simulink model "c00017M_harness"  (R2018a)
settings: Solver=ode3  StartTime=0.0  StopTime=10.0  RelTol=1e-3  EnableMultiTasking=on
undefined symbols (not defined in the file): b, DiscIntNeverNeededParam, J, K, L, PosMinimaW3, PosMinimaW4, R, sigbuilder_block
(part 3 of 68)

== system c00017M_harness/Eval134 ==
  In1 : Inport
  In2 : Inport  Port=2
  In3 : Inport  Port=3
  In4 : Inport  Port=4
  Data Type Conversion{,1..3} (4 alike) : DataTypeConversion
  Memory{1..4} (4 alike) : Memory  InitialCondition=1
  MinMax : MinMax  Inputs=4
  MinMax{1..4} (4 alike) : MinMax  Inputs=2
  ROOut{1..4} (4 alike) : RelationalOperator  Operator===  OutDataTypeStr=boolean  RndMeth=Simplest
  Out1 : Outport
  wires:
  Data Type Conversion3/1 -> MinMax4/1
  Data Type Conversion2/1 -> MinMax3/1
  Data Type Conversion1/1 -> MinMax2/1
  Data Type Conversion/1 -> MinMax1/1
  MinMax1/1 -> Memory1/1, MinMax/1
  ROOut4/1 -> Data Type Conversion3/1
  MinMax2/1 -> Memory2/1, MinMax/2
  ROOut1/1 -> Data Type Conversion/1
  Memory2/1 -> MinMax2/2
  Memory4/1 -> MinMax4/2
  Memory3/1 -> MinMax3/2
  ROOut2/1 -> Data Type Conversion1/1
  ROOut3/1 -> Data Type Conversion2/1
  MinMax3/1 -> Memory3/1, MinMax/3
  MinMax4/1 -> Memory4/1, MinMax/4
  Memory1/1 -> MinMax1/2
  [out4] -> ROOut4/2
  In4/1 -> ROOut4/1
  [out2] -> ROOut2/2
  In1/1 -> ROOut1/1
  In2/1 -> ROOut2/1
  [out1] -> ROOut1/2
  In3/1 -> ROOut3/1
  [out3] -> ROOut3/2
  MinMax/1 -> Out1/1

== system c00017M_harness/Eval135 ==
  In1 : Inport
  In2 : Inport  Port=2
  In3 : Inport  Port=3
  In4 : Inport  Port=4
  Data Type Conversion{,1..3} (4 alike) : DataTypeConversion
  Memory{1..4} (4 alike) : Memory  InitialCondition=1
  MinMax : MinMax  Inputs=4
  MinMax{1..4} (4 alike) : MinMax  Inputs=2
  ROOut{1..4} (4 alike) : RelationalOperator  Operator===  OutDataTypeStr=boolean  RndMeth=Simplest
  Out1 : Outport
  wires:
  Data Type Conversion3/1 -> MinMax4/1
  Data Type Conversion2/1 -> MinMax3/1
  Data Type Conversion1/1 -> MinMax2/1
  Data Type Conversion/1 -> MinMax1/1
  MinMax1/1 -> Memory1/1, MinMax/1
  ROOut4/1 -> Data Type Conversion3/1
  MinMax2/1 -> Memory2/1, MinMax/2
  ROOut1/1 -> Data Type Conversion/1
  Memory2/1 -> MinMax2/2
  Memory4/1 -> MinMax4/2
  Memory3/1 -> MinMax3/2
  ROOut2/1 -> Data Type Conversion1/1
  ROOut3/1 -> Data Type Conversion2/1
  MinMax3/1 -> Memory3/1, MinMax/3
  MinMax4/1 -> Memory4/1, MinMax/4
  Memory1/1 -> MinMax1/2
  [out4] -> ROOut4/2
  In4/1 -> ROOut4/1
  [out2] -> ROOut2/2
  In1/1 -> ROOut1/1
  In2/1 -> ROOut2/1
  [out1] -> ROOut1/2
  In3/1 -> ROOut3/1
  [out3] -> ROOut3/2
  MinMax/1 -> Out1/1

== system c00017M_harness/Eval136 ==
  In1 : Inport
  In2 : Inport  Port=2
  In3 : Inport  Port=3
  In4 : Inport  Port=4
  Data Type Conversion{,1..3} (4 alike) : DataTypeConversion
  Memory{1..4} (4 alike) : Memory  InitialCondition=1
  MinMax : MinMax  Inputs=4
  MinMax{1..4} (4 alike) : MinMax  Inputs=2
  ROOut{1..4} (4 alike) : RelationalOperator  Operator===  OutDataTypeStr=boolean  RndMeth=Simplest
  Out1 : Outport
  wires:
  Data Type Conversion3/1 -> MinMax4/1
  Data Type Conversion2/1 -> MinMax3/1
  Data Type Conversion1/1 -> MinMax2/1
  Data Type Conversion/1 -> MinMax1/1
  MinMax1/1 -> Memory1/1, MinMax/1
  ROOut4/1 -> Data Type Conversion3/1
  MinMax2/1 -> Memory2/1, MinMax/2
  ROOut1/1 -> Data Type Conversion/1
  Memory2/1 -> MinMax2/2
  Memory4/1 -> MinMax4/2
  Memory3/1 -> MinMax3/2
  ROOut2/1 -> Data Type Conversion1/1
  ROOut3/1 -> Data Type Conversion2/1
  MinMax3/1 -> Memory3/1, MinMax/3
  MinMax4/1 -> Memory4/1, MinMax/4
  Memory1/1 -> MinMax1/2
  [out4] -> ROOut4/2
  In4/1 -> ROOut4/1
  [out2] -> ROOut2/2
  In1/1 -> ROOut1/1
  In2/1 -> ROOut2/1
  [out1] -> ROOut1/2
  In3/1 -> ROOut3/1
  [out3] -> ROOut3/2
  MinMax/1 -> Out1/1

== system c00017M_harness/Eval137 ==
  In1 : Inport
  In2 : Inport  Port=2
  In3 : Inport  Port=3
  In4 : Inport  Port=4
  Data Type Conversion{,1..3} (4 alike) : DataTypeConversion
  Memory{1..4} (4 alike) : Memory  InitialCondition=1
  MinMax : MinMax  Inputs=4
  MinMax{1..4} (4 alike) : MinMax  Inputs=2
  ROOut{1..4} (4 alike) : RelationalOperator  Operator===  OutDataTypeStr=boolean  RndMeth=Simplest
  Out1 : Outport
  wires:
  Data Type Conversion3/1 -> MinMax4/1
  Data Type Conversion2/1 -> MinMax3/1
  Data Type Conversion1/1 -> MinMax2/1
  Data Type Conversion/1 -> MinMax1/1
  MinMax1/1 -> Memory1/1, MinMax/1
  ROOut4/1 -> Data Type Conversion3/1
  MinMax2/1 -> Memory2/1, MinMax/2
  ROOut1/1 -> Data Type Conversion/1
  Memory2/1 -> MinMax2/2
  Memory4/1 -> MinMax4/2
  Memory3/1 -> MinMax3/2
  ROOut2/1 -> Data Type Conversion1/1
  ROOut3/1 -> Data Type Conversion2/1
  MinMax3/1 -> Memory3/1, MinMax/3
  MinMax4/1 -> Memory4/1, MinMax/4
  Memory1/1 -> MinMax1/2
  [out4] -> ROOut4/2
  In4/1 -> ROOut4/1
  [out2] -> ROOut2/2
  In1/1 -> ROOut1/1
  In2/1 -> ROOut2/1
  [out1] -> ROOut1/2
  In3/1 -> ROOut3/1
  [out3] -> ROOut3/2
  MinMax/1 -> Out1/1

== system c00017M_harness/Eval138 ==
  In1 : Inport
  In2 : Inport  Port=2
  In3 : Inport  Port=3
  In4 : Inport  Port=4
  Data Type Conversion{,1..3} (4 alike) : DataTypeConversion
  Memory{1..4} (4 alike) : Memory  InitialCondition=1
  MinMax : MinMax  Inputs=4
  MinMax{1..4} (4 alike) : MinMax  Inputs=2
  ROOut{1..4} (4 alike) : RelationalOperator  Operator===  OutDataTypeStr=boolean  RndMeth=Simplest
  Out1 : Outport
  wires:
  Data Type Conversion3/1 -> MinMax4/1
  Data Type Conversion2/1 -> MinMax3/1
  Data Type Conversion1/1 -> MinMax2/1
  Data Type Conversion/1 -> MinMax1/1
  MinMax1/1 -> Memory1/1, MinMax/1
  ROOut4/1 -> Data Type Conversion3/1
  MinMax2/1 -> Memory2/1, MinMax/2
  ROOut1/1 -> Data Type Conversion/1
  Memory2/1 -> MinMax2/2
  Memory4/1 -> MinMax4/2
  Memory3/1 -> MinMax3/2
  ROOut2/1 -> Data Type Conversion1/1
  ROOut3/1 -> Data Type Conversion2/1
  MinMax3/1 -> Memory3/1, MinMax/3
  MinMax4/1 -> Memory4/1, MinMax/4
  Memory1/1 -> MinMax1/2
  [out4] -> ROOut4/2
  In4/1 -> ROOut4/1
  [out2] -> ROOut2/2
  In1/1 -> ROOut1/1
  In2/1 -> ROOut2/1
  [out1] -> ROOut1/2
  In3/1 -> ROOut3/1
  [out3] -> ROOut3/2
  MinMax/1 -> Out1/1

== system c00017M_harness/Eval139 ==
  In1 : Inport
  In2 : Inport  Port=2
  In3 : Inport  Port=3
  In4 : Inport  Port=4
  Data Type Conversion{,1..3} (4 alike) : DataTypeConversion
  Memory{1..4} (4 alike) : Memory  InitialCondition=1
  MinMax : MinMax  Inputs=4
  MinMax{1..4} (4 alike) : MinMax  Inputs=2
  ROOut{1..4} (4 alike) : RelationalOperator  Operator===  OutDataTypeStr=boolean  RndMeth=Simplest
  Out1 : Outport
  wires:
  Data Type Conversion3/1 -> MinMax4/1
  Data Type Conversion2/1 -> MinMax3/1
  Data Type Conversion1/1 -> MinMax2/1
  Data Type Conversion/1 -> MinMax1/1
  MinMax1/1 -> Memory1/1, MinMax/1
  ROOut4/1 -> Data Type Conversion3/1
  MinMax2/1 -> Memory2/1, MinMax/2
  ROOut1/1 -> Data Type Conversion/1
  Memory2/1 -> MinMax2/2
  Memory4/1 -> MinMax4/2
  Memory3/1 -> MinMax3/2
  ROOut2/1 -> Data Type Conversion1/1
  ROOut3/1 -> Data Type Conversion2/1
  MinMax3/1 -> Memory3/1, MinMax/3
  MinMax4/1 -> Memory4/1, MinMax/4
  Memory1/1 -> MinMax1/2
  [out4] -> ROOut4/2
  In4/1 -> ROOut4/1
  [out2] -> ROOut2/2
  In1/1 -> ROOut1/1
  In2/1 -> ROOut2/1
  [out1] -> ROOut1/2
  In3/1 -> ROOut3/1
  [out3] -> ROOut3/2
  MinMax/1 -> Out1/1

== system c00017M_harness/Eval14 ==
  In1 : Inport
  In2 : Inport  Port=2
  In3 : Inport  Port=3
  In4 : Inport  Port=4
  Data Type Conversion{,1..3} (4 alike) : DataTypeConversion
  Memory{1..4} (4 alike) : Memory  InitialCondition=1
  MinMax : MinMax  Inputs=4
  MinMax{1..4} (4 alike) : MinMax  Inputs=2
  ROOut{1..4} (4 alike) : RelationalOperator  Operator===  OutDataTypeStr=boolean  RndMeth=Simplest
  Out1 : Outport
  wires:
  Data Type Conversion3/1 -> MinMax4/1
  Data Type Conversion2/1 -> MinMax3/1
  Data Type Conversion1/1 -> MinMax2/1
  Data Type Conversion/1 -> MinMax1/1
  MinMax1/1 -> Memory1/1, MinMax/1
  ROOut4/1 -> Data Type Conversion3/1
  MinMax2/1 -> Memory2/1, MinMax/2
  ROOut1/1 -> Data Type Conversion/1
  Memory2/1 -> MinMax2/2
  Memory4/1 -> MinMax4/2
  Memory3/1 -> MinMax3/2
  ROOut2/1 -> Data Type Conversion1/1
  ROOut3/1 -> Data Type Conversion2/1
  MinMax3/1 -> Memory3/1, MinMax/3
  MinMax4/1 -> Memory4/1, MinMax/4
  Memory1/1 -> MinMax1/2
  [out4] -> ROOut4/2
  In4/1 -> ROOut4/1
  [out2] -> ROOut2/2
  In1/1 -> ROOut1/1
  In2/1 -> ROOut2/1
  [out1] -> ROOut1/2
  In3/1 -> ROOut3/1
  [out3] -> ROOut3/2
  MinMax/1 -> Out1/1

== system c00017M_harness/Eval140 ==
  In1 : Inport
  In2 : Inport  Port=2
  In3 : Inport  Port=3
  In4 : Inport  Port=4
  Data Type Conversion{,1..3} (4 alike) : DataTypeConversion
  Memory{1..4} (4 alike) : Memory  InitialCondition=1
  MinMax : MinMax  Inputs=4
  MinMax{1..4} (4 alike) : MinMax  Inputs=2
  ROOut{1..4} (4 alike) : RelationalOperator  Operator===  OutDataTypeStr=boolean  RndMeth=Simplest
  Out1 : Outport
  wires:
  Data Type Conversion3/1 -> MinMax4/1
  Data Type Conversion2/1 -> MinMax3/1
  Data Type Conversion1/1 -> MinMax2/1
  Data Type Conversion/1 -> MinMax1/1
  MinMax1/1 -> Memory1/1, MinMax/1
  ROOut4/1 -> Data Type Conversion3/1
  MinMax2/1 -> Memory2/1, MinMax/2
  ROOut1/1 -> Data Type Conversion/1
  Memory2/1 -> MinMax2/2
  Memory4/1 -> MinMax4/2
  Memory3/1 -> MinMax3/2
  ROOut2/1 -> Data Type Conversion1/1
  ROOut3/1 -> Data Type Conversion2/1
  MinMax3/1 -> Memory3/1, MinMax/3
  MinMax4/1 -> Memory4/1, MinMax/4
  Memory1/1 -> MinMax1/2
  [out4] -> ROOut4/2
  In4/1 -> ROOut4/1
  [out2] -> ROOut2/2
  In1/1 -> ROOut1/1
  In2/1 -> ROOut2/1
  [out1] -> ROOut1/2
  In3/1 -> ROOut3/1
  [out3] -> ROOut3/2
  MinMax/1 -> Out1/1

== system c00017M_harness/Eval141 ==
  In1 : Inport
  In2 : Inport  Port=2
  In3 : Inport  Port=3
  In4 : Inport  Port=4
  Data Type Conversion{,1..3} (4 alike) : DataTypeConversion
  Memory{1..4} (4 alike) : Memory  InitialCondition=1
  MinMax : MinMax  Inputs=4
  MinMax{1..4} (4 alike) : MinMax  Inputs=2
  ROOut{1..4} (4 alike) : RelationalOperator  Operator===  OutDataTypeStr=boolean  RndMeth=Simplest
  Out1 : Outport
  wires:
  Data Type Conversion3/1 -> MinMax4/1
  Data Type Conversion2/1 -> MinMax3/1
  Data Type Conversion1/1 -> MinMax2/1
  Data Type Conversion/1 -> MinMax1/1
  MinMax1/1 -> Memory1/1, MinMax/1
  ROOut4/1 -> Data Type Conversion3/1
  MinMax2/1 -> Memory2/1, MinMax/2
  ROOut1/1 -> Data Type Conversion/1
  Memory2/1 -> MinMax2/2
  Memory4/1 -> MinMax4/2
  Memory3/1 -> MinMax3/2
  ROOut2/1 -> Data Type Conversion1/1
  ROOut3/1 -> Data Type Conversion2/1
  MinMax3/1 -> Memory3/1, MinMax/3
  MinMax4/1 -> Memory4/1, MinMax/4
  Memory1/1 -> MinMax1/2
  [out4] -> ROOut4/2
  In4/1 -> ROOut4/1
  [out2] -> ROOut2/2
  In1/1 -> ROOut1/1
  In2/1 -> ROOut2/1
  [out1] -> ROOut1/2
  In3/1 -> ROOut3/1
  [out3] -> ROOut3/2
  MinMax/1 -> Out1/1

== system c00017M_harness/Eval142 ==
  In1 : Inport
  In2 : Inport  Port=2
  In3 : Inport  Port=3
  In4 : Inport  Port=4
  Data Type Conversion{,1..3} (4 alike) : DataTypeConversion
  Memory{1..4} (4 alike) : Memory  InitialCondition=1
  MinMax : MinMax  Inputs=4
  MinMax{1..4} (4 alike) : MinMax  Inputs=2
  ROOut{1..4} (4 alike) : RelationalOperator  Operator===  OutDataTypeStr=boolean  RndMeth=Simplest
  Out1 : Outport
  wires:
  Data Type Conversion3/1 -> MinMax4/1
  Data Type Conversion2/1 -> MinMax3/1
  Data Type Conversion1/1 -> MinMax2/1
  Data Type Conversion/1 -> MinMax1/1
  MinMax1/1 -> Memory1/1, MinMax/1
  ROOut4/1 -> Data Type Conversion3/1
  MinMax2/1 -> Memory2/1, MinMax/2
  ROOut1/1 -> Data Type Conversion/1
  Memory2/1 -> MinMax2/2
  Memory4/1 -> MinMax4/2
  Memory3/1 -> MinMax3/2
  ROOut2/1 -> Data Type Conversion1/1
  ROOut3/1 -> Data Type Conversion2/1
  MinMax3/1 -> Memory3/1, MinMax/3
  MinMax4/1 -> Memory4/1, MinMax/4
  Memory1/1 -> MinMax1/2
  [out4] -> ROOut4/2
  In4/1 -> ROOut4/1
  [out2] -> ROOut2/2
  In1/1 -> ROOut1/1
  In2/1 -> ROOut2/1
  [out1] -> ROOut1/2
  In3/1 -> ROOut3/1
  [out3] -> ROOut3/2
  MinMax/1 -> Out1/1

== system c00017M_harness/Eval143 ==
  In1 : Inport
  In2 : Inport  Port=2
  In3 : Inport  Port=3
  In4 : Inport  Port=4
  Data Type Conversion{,1..3} (4 alike) : DataTypeConversion
  Memory{1..4} (4 alike) : Memory  InitialCondition=1
  MinMax : MinMax  Inputs=4
  MinMax{1..4} (4 alike) : MinMax  Inputs=2
  ROOut{1..4} (4 alike) : RelationalOperator  Operator===  OutDataTypeStr=boolean  RndMeth=Simplest
  Out1 : Outport
  wires:
  Data Type Conversion3/1 -> MinMax4/1
  Data Type Conversion2/1 -> MinMax3/1
  Data Type Conversion1/1 -> MinMax2/1
  Data Type Conversion/1 -> MinMax1/1
  MinMax1/1 -> Memory1/1, MinMax/1
  ROOut4/1 -> Data Type Conversion3/1
  MinMax2/1 -> Memory2/1, MinMax/2
  ROOut1/1 -> Data Type Conversion/1
  Memory2/1 -> MinMax2/2
  Memory4/1 -> MinMax4/2
  Memory3/1 -> MinMax3/2
  ROOut2/1 -> Data Type Conversion1/1
  ROOut3/1 -> Data Type Conversion2/1
  MinMax3/1 -> Memory3/1, MinMax/3
  MinMax4/1 -> Memory4/1, MinMax/4
  Memory1/1 -> MinMax1/2
  [out4] -> ROOut4/2
  In4/1 -> ROOut4/1
  [out2] -> ROOut2/2
  In1/1 -> ROOut1/1
  In2/1 -> ROOut2/1
  [out1] -> ROOut1/2
  In3/1 -> ROOut3/1
  [out3] -> ROOut3/2
  MinMax/1 -> Out1/1

== system c00017M_harness/Eval144 ==
  In1 : Inport
  In2 : Inport  Port=2
  In3 : Inport  Port=3
  In4 : Inport  Port=4
  Data Type Conversion{,1..3} (4 alike) : DataTypeConversion
  Memory{1..4} (4 alike) : Memory  InitialCondition=1
  MinMax : MinMax  Inputs=4
  MinMax{1..4} (4 alike) : MinMax  Inputs=2
  ROOut{1..4} (4 alike) : RelationalOperator  Operator===  OutDataTypeStr=boolean  RndMeth=Simplest
  Out1 : Outport
  wires:
  Data Type Conversion3/1 -> MinMax4/1
  Data Type Conversion2/1 -> MinMax3/1
  Data Type Conversion1/1 -> MinMax2/1
  Data Type Conversion/1 -> MinMax1/1
  MinMax1/1 -> Memory1/1, MinMax/1
  ROOut4/1 -> Data Type Conversion3/1
  MinMax2/1 -> Memory2/1, MinMax/2
  ROOut1/1 -> Data Type Conversion/1
  Memory2/1 -> MinMax2/2
  Memory4/1 -> MinMax4/2
  Memory3/1 -> MinMax3/2
  ROOut2/1 -> Data Type Conversion1/1
  ROOut3/1 -> Data Type Conversion2/1
  MinMax3/1 -> Memory3/1, MinMax/3
  MinMax4/1 -> Memory4/1, MinMax/4
  Memory1/1 -> MinMax1/2
  [out4] -> ROOut4/2
  In4/1 -> ROOut4/1
  [out2] -> ROOut2/2
  In1/1 -> ROOut1/1
  In2/1 -> ROOut2/1
  [out1] -> ROOut1/2
  In3/1 -> ROOut3/1
  [out3] -> ROOut3/2
  MinMax/1 -> Out1/1

== system c00017M_harness/Eval145 ==
  In1 : Inport
  In2 : Inport  Port=2
  In3 : Inport  Port=3
  In4 : Inport  Port=4
  Data Type Conversion{,1..3} (4 alike) : DataTypeConversion
  Memory{1..4} (4 alike) : Memory  InitialCondition=1
  MinMax : MinMax  Inputs=4
  MinMax{1..4} (4 alike) : MinMax  Inputs=2
  ROOut{1..4} (4 alike) : RelationalOperator  Operator===  OutDataTypeStr=boolean  RndMeth=Simplest
  Out1 : Outport
  wires:
  Data Type Conversion3/1 -> MinMax4/1
  Data Type Conversion2/1 -> MinMax3/1
  Data Type Conversion1/1 -> MinMax2/1
  Data Type Conversion/1 -> MinMax1/1
  MinMax1/1 -> Memory1/1, MinMax/1
  ROOut4/1 -> Data Type Conversion3/1
  MinMax2/1 -> Memory2/1, MinMax/2
  ROOut1/1 -> Data Type Conversion/1
  Memory2/1 -> MinMax2/2
  Memory4/1 -> MinMax4/2
  Memory3/1 -> MinMax3/2
  ROOut2/1 -> Data Type Conversion1/1
  ROOut3/1 -> Data Type Conversion2/1
  MinMax3/1 -> Memory3/1, MinMax/3
  MinMax4/1 -> Memory4/1, MinMax/4
  Memory1/1 -> MinMax1/2
  [out4] -> ROOut4/2
  In4/1 -> ROOut4/1
  [out2] -> ROOut2/2
  In1/1 -> ROOut1/1
  In2/1 -> ROOut2/1
  [out1] -> ROOut1/2
  In3/1 -> ROOut3/1
  [out3] -> ROOut3/2
  MinMax/1 -> Out1/1

== system c00017M_harness/Eval146 ==
  In1 : Inport
  In2 : Inport  Port=2
  In3 : Inport  Port=3
  In4 : Inport  Port=4
  Data Type Conversion{,1..3} (4 alike) : DataTypeConversion
  Memory{1..4} (4 alike) : Memory  InitialCondition=1
  MinMax : MinMax  Inputs=4
  MinMax{1..4} (4 alike) : MinMax  Inputs=2
  ROOut{1..4} (4 alike) : RelationalOperator  Operator===  OutDataTypeStr=boolean  RndMeth=Simplest
  Out1 : Outport
  wires:
  Data Type Conversion3/1 -> MinMax4/1
  Data Type Conversion2/1 -> MinMax3/1
  Data Type Conversion1/1 -> MinMax2/1
  Data Type Conversion/1 -> MinMax1/1
  MinMax1/1 -> Memory1/1, MinMax/1
  ROOut4/1 -> Data Type Conversion3/1
  MinMax2/1 -> Memory2/1, MinMax/2
  ROOut1/1 -> Data Type Conversion/1
  Memory2/1 -> MinMax2/2
  Memory4/1 -> MinMax4/2
  Memory3/1 -> MinMax3/2
  ROOut2/1 -> Data Type Conversion1/1
  ROOut3/1 -> Data Type Conversion2/1
  MinMax3/1 -> Memory3/1, MinMax/3
  MinMax4/1 -> Memory4/1, MinMax/4
  Memory1/1 -> MinMax1/2
  [out4] -> ROOut4/2
  In4/1 -> ROOut4/1
  [out2] -> ROOut2/2
  In1/1 -> ROOut1/1
  In2/1 -> ROOut2/1
  [out1] -> ROOut1/2
  In3/1 -> ROOut3/1
  [out3] -> ROOut3/2
  MinMax/1 -> Out1/1

== system c00017M_harness/Eval147 ==
  In1 : Inport
  In2 : Inport  Port=2
  In3 : Inport  Port=3
  In4 : Inport  Port=4
  Data Type Conversion{,1..3} (4 alike) : DataTypeConversion
  Memory{1..4} (4 alike) : Memory  InitialCondition=1
  MinMax : MinMax  Inputs=4
  MinMax{1..4} (4 alike) : MinMax  Inputs=2
  ROOut{1..4} (4 alike) : RelationalOperator  Operator===  OutDataTypeStr=boolean  RndMeth=Simplest
  Out1 : Outport
  wires:
  Data Type Conversion3/1 -> MinMax4/1
  Data Type Conversion2/1 -> MinMax3/1
  Data Type Conversion1/1 -> MinMax2/1
  Data Type Conversion/1 -> MinMax1/1
  MinMax1/1 -> Memory1/1, MinMax/1
  ROOut4/1 -> Data Type Conversion3/1
  MinMax2/1 -> Memory2/1, MinMax/2
  ROOut1/1 -> Data Type Conversion/1
  Memory2/1 -> MinMax2/2
  Memory4/1 -> MinMax4/2
  Memory3/1 -> MinMax3/2
  ROOut2/1 -> Data Type Conversion1/1
  ROOut3/1 -> Data Type Conversion2/1
  MinMax3/1 -> Memory3/1, MinMax/3
  MinMax4/1 -> Memory4/1, MinMax/4
  Memory1/1 -> MinMax1/2
  [out4] -> ROOut4/2
  In4/1 -> ROOut4/1
  [out2] -> ROOut2/2
  In1/1 -> ROOut1/1
  In2/1 -> ROOut2/1
  [out1] -> ROOut1/2
  In3/1 -> ROOut3/1
  [out3] -> ROOut3/2
  MinMax/1 -> Out1/1

== system c00017M_harness/Eval148 ==
  In1 : Inport
  In2 : Inport  Port=2
  In3 : Inport  Port=3
  In4 : Inport  Port=4
  Data Type Conversion{,1..3} (4 alike) : DataTypeConversion
  Memory{1..4} (4 alike) : Memory  InitialCondition=1
  MinMax : MinMax  Inputs=4
  MinMax{1..4} (4 alike) : MinMax  Inputs=2
  ROOut{1..4} (4 alike) : RelationalOperator  Operator===  OutDataTypeStr=boolean  RndMeth=Simplest
  Out1 : Outport
  wires:
  Data Type Conversion3/1 -> MinMax4/1
  Data Type Conversion2/1 -> MinMax3/1
  Data Type Conversion1/1 -> MinMax2/1
  Data Type Conversion/1 -> MinMax1/1
  MinMax1/1 -> Memory1/1, MinMax/1
  ROOut4/1 -> Data Type Conversion3/1
  MinMax2/1 -> Memory2/1, MinMax/2
  ROOut1/1 -> Data Type Conversion/1
  Memory2/1 -> MinMax2/2
  Memory4/1 -> MinMax4/2
  Memory3/1 -> MinMax3/2
  ROOut2/1 -> Data Type Conversion1/1
  ROOut3/1 -> Data Type Conversion2/1
  MinMax3/1 -> Memory3/1, MinMax/3
  MinMax4/1 -> Memory4/1, MinMax/4
  Memory1/1 -> MinMax1/2
  [out4] -> ROOut4/2
  In4/1 -> ROOut4/1
  [out2] -> ROOut2/2
  In1/1 -> ROOut1/1
  In2/1 -> ROOut2/1
  [out1] -> ROOut1/2
  In3/1 -> ROOut3/1
  [out3] -> ROOut3/2
  MinMax/1 -> Out1/1

== system c00017M_harness/Eval149 ==
  In1 : Inport
  In2 : Inport  Port=2
  In3 : Inport  Port=3
  In4 : Inport  Port=4
  Data Type Conversion{,1..3} (4 alike) : DataTypeConversion
  Memory{1..4} (4 alike) : Memory  InitialCondition=1
  MinMax : MinMax  Inputs=4
  MinMax{1..4} (4 alike) : MinMax  Inputs=2
  ROOut{1..4} (4 alike) : RelationalOperator  Operator===  OutDataTypeStr=boolean  RndMeth=Simplest
  Out1 : Outport
  wires:
  Data Type Conversion3/1 -> MinMax4/1
  Data Type Conversion2/1 -> MinMax3/1
  Data Type Conversion1/1 -> MinMax2/1
  Data Type Conversion/1 -> MinMax1/1
  MinMax1/1 -> Memory1/1, MinMax/1
  ROOut4/1 -> Data Type Conversion3/1
  MinMax2/1 -> Memory2/1, MinMax/2
  ROOut1/1 -> Data Type Conversion/1
  Memory2/1 -> MinMax2/2
  Memory4/1 -> MinMax4/2
  Memory3/1 -> MinMax3/2
  ROOut2/1 -> Data Type Conversion1/1
  ROOut3/1 -> Data Type Conversion2/1
  MinMax3/1 -> Memory3/1, MinMax/3
  MinMax4/1 -> Memory4/1, MinMax/4
  Memory1/1 -> MinMax1/2
  [out4] -> ROOut4/2
  In4/1 -> ROOut4/1
  [out2] -> ROOut2/2
  In1/1 -> ROOut1/1
  In2/1 -> ROOut2/1
  [out1] -> ROOut1/2
  In3/1 -> ROOut3/1
  [out3] -> ROOut3/2
  MinMax/1 -> Out1/1

== system c00017M_harness/Eval15 ==
  In1 : Inport
  In2 : Inport  Port=2
  In3 : Inport  Port=3
  In4 : Inport  Port=4
  Data Type Conversion{,1..3} (4 alike) : DataTypeConversion
  Memory{1..4} (4 alike) : Memory  InitialCondition=1
  MinMax : MinMax  Inputs=4
  MinMax{1..4} (4 alike) : MinMax  Inputs=2
  ROOut{1..4} (4 alike) : RelationalOperator  Operator===  OutDataTypeStr=boolean  RndMeth=Simplest
  Out1 : Outport
  wires:
  Data Type Conversion3/1 -> MinMax4/1
  Data Type Conversion2/1 -> MinMax3/1
  Data Type Conversion1/1 -> MinMax2/1
  Data Type Conversion/1 -> MinMax1/1
  MinMax1/1 -> Memory1/1, MinMax/1
  ROOut4/1 -> Data Type Conversion3/1
  MinMax2/1 -> Memory2/1, MinMax/2
  ROOut1/1 -> Data Type Conversion/1
  Memory2/1 -> MinMax2/2
  Memory4/1 -> MinMax4/2
  Memory3/1 -> MinMax3/2
  ROOut2/1 -> Data Type Conversion1/1
  ROOut3/1 -> Data Type Conversion2/1
  MinMax3/1 -> Memory3/1, MinMax/3
  MinMax4/1 -> Memory4/1, MinMax/4
  Memory1/1 -> MinMax1/2
  [out4] -> ROOut4/2
  In4/1 -> ROOut4/1
  [out2] -> ROOut2/2
  In1/1 -> ROOut1/1
  In2/1 -> ROOut2/1
  [out1] -> ROOut1/2
  In3/1 -> ROOut3/1
  [out3] -> ROOut3/2
  MinMax/1 -> Out1/1

== system c00017M_harness/Eval150 ==
  In1 : Inport
  In2 : Inport  Port=2
  In3 : Inport  Port=3
  In4 : Inport  Port=4
  Data Type Conversion{,1..3} (4 alike) : DataTypeConversion
  Memory{1..4} (4 alike) : Memory  InitialCondition=1
  MinMax : MinMax  Inputs=4
  MinMax{1..4} (4 alike) : MinMax  Inputs=2
  ROOut{1..4} (4 alike) : RelationalOperator  Operator===  OutDataTypeStr=boolean  RndMeth=Simplest
  Out1 : Outport
  wires:
  Data Type Conversion3/1 -> MinMax4/1
  Data Type Conversion2/1 -> MinMax3/1
  Data Type Conversion1/1 -> MinMax2/1
  Data Type Conversion/1 -> MinMax1/1
  MinMax1/1 -> Memory1/1, MinMax/1
  ROOut4/1 -> Data Type Conversion3/1
  MinMax2/1 -> Memory2/1, MinMax/2
  ROOut1/1 -> Data Type Conversion/1
  Memory2/1 -> MinMax2/2
  Memory4/1 -> MinMax4/2
  Memory3/1 -> MinMax3/2
  ROOut2/1 -> Data Type Conversion1/1
  ROOut3/1 -> Data Type Conversion2/1
  MinMax3/1 -> Memory3/1, MinMax/3
  MinMax4/1 -> Memory4/1, MinMax/4
  Memory1/1 -> MinMax1/2
  [out4] -> ROOut4/2
  In4/1 -> ROOut4/1
  [out2] -> ROOut2/2
  In1/1 -> ROOut1/1
  In2/1 -> ROOut2/1
  [out1] -> ROOut1/2
  In3/1 -> ROOut3/1
  [out3] -> ROOut3/2
  MinMax/1 -> Out1/1

== system c00017M_harness/Eval151 ==
  In1 : Inport
  In2 : Inport  Port=2
  In3 : Inport  Port=3
  In4 : Inport  Port=4
  Data Type Conversion{,1..3} (4 alike) : DataTypeConversion
  Memory{1..4} (4 alike) : Memory  InitialCondition=1
  MinMax : MinMax  Inputs=4
  MinMax{1..4} (4 alike) : MinMax  Inputs=2
  ROOut{1..4} (4 alike) : RelationalOperator  Operator===  OutDataTypeStr=boolean  RndMeth=Simplest
  Out1 : Outport
  wires:
  Data Type Conversion3/1 -> MinMax4/1
  Data Type Conversion2/1 -> MinMax3/1
  Data Type Conversion1/1 -> MinMax2/1
  Data Type Conversion/1 -> MinMax1/1
  MinMax1/1 -> Memory1/1, MinMax/1
  ROOut4/1 -> Data Type Conversion3/1
  MinMax2/1 -> Memory2/1, MinMax/2
  ROOut1/1 -> Data Type Conversion/1
  Memory2/1 -> MinMax2/2
  Memory4/1 -> MinMax4/2
  Memory3/1 -> MinMax3/2
  ROOut2/1 -> Data Type Conversion1/1
  ROOut3/1 -> Data Type Conversion2/1
  MinMax3/1 -> Memory3/1, MinMax/3
  MinMax4/1 -> Memory4/1, MinMax/4
  Memory1/1 -> MinMax1/2
  [out4] -> ROOut4/2
  In4/1 -> ROOut4/1
  [out2] -> ROOut2/2
  In1/1 -> ROOut1/1
  In2/1 -> ROOut2/1
  [out1] -> ROOut1/2
  In3/1 -> ROOut3/1
  [out3] -> ROOut3/2
  MinMax/1 -> Out1/1

== system c00017M_harness/Eval152 ==
  In1 : Inport
  In2 : Inport  Port=2
  In3 : Inport  Port=3
  In4 : Inport  Port=4
  Data Type Conversion{,1..3} (4 alike) : DataTypeConversion
  Memory{1..4} (4 alike) : Memory  InitialCondition=1
  MinMax : MinMax  Inputs=4
  MinMax{1..4} (4 alike) : MinMax  Inputs=2
  ROOut{1..4} (4 alike) : RelationalOperator  Operator===  OutDataTypeStr=boolean  RndMeth=Simplest
  Out1 : Outport
  wires:
  Data Type Conversion3/1 -> MinMax4/1
  Data Type Conversion2/1 -> MinMax3/1
  Data Type Conversion1/1 -> MinMax2/1
  Data Type Conversion/1 -> MinMax1/1
  MinMax1/1 -> Memory1/1, MinMax/1
  ROOut4/1 -> Data Type Conversion3/1
  MinMax2/1 -> Memory2/1, MinMax/2
  ROOut1/1 -> Data Type Conversion/1
  Memory2/1 -> MinMax2/2
  Memory4/1 -> MinMax4/2
  Memory3/1 -> MinMax3/2
  ROOut2/1 -> Data Type Conversion1/1
  ROOut3/1 -> Data Type Conversion2/1
  MinMax3/1 -> Memory3/1, MinMax/3
  MinMax4/1 -> Memory4/1, MinMax/4
  Memory1/1 -> MinMax1/2
  [out4] -> ROOut4/2
  In4/1 -> ROOut4/1
  [out2] -> ROOut2/2
  In1/1 -> ROOut1/1
  In2/1 -> ROOut2/1
  [out1] -> ROOut1/2
  In3/1 -> ROOut3/1
  [out3] -> ROOut3/2
  MinMax/1 -> Out1/1

== system c00017M_harness/Eval153 ==
  In1 : Inport
  In2 : Inport  Port=2
  In3 : Inport  Port=3
  In4 : Inport  Port=4
  Data Type Conversion{,1..3} (4 alike) : DataTypeConversion
  Memory{1..4} (4 alike) : Memory  InitialCondition=1
  MinMax : MinMax  Inputs=4
  MinMax{1..4} (4 alike) : MinMax  Inputs=2
  ROOut{1..4} (4 alike) : RelationalOperator  Operator===  OutDataTypeStr=boolean  RndMeth=Simplest
  Out1 : Outport
  wires:
  Data Type Conversion3/1 -> MinMax4/1
  Data Type Conversion2/1 -> MinMax3/1
  Data Type Conversion1/1 -> MinMax2/1
  Data Type Conversion/1 -> MinMax1/1
  MinMax1/1 -> Memory1/1, MinMax/1
  ROOut4/1 -> Data Type Conversion3/1
  MinMax2/1 -> Memory2/1, MinMax/2
  ROOut1/1 -> Data Type Conversion/1
  Memory2/1 -> MinMax2/2
  Memory4/1 -> MinMax4/2
  Memory3/1 -> MinMax3/2
  ROOut2/1 -> Data Type Conversion1/1
  ROOut3/1 -> Data Type Conversion2/1
  MinMax3/1 -> Memory3/1, MinMax/3
  MinMax4/1 -> Memory4/1, MinMax/4
  Memory1/1 -> MinMax1/2
  [out4] -> ROOut4/2
  In4/1 -> ROOut4/1
  [out2] -> ROOut2/2
  In1/1 -> ROOut1/1
  In2/1 -> ROOut2/1
  [out1] -> ROOut1/2
  In3/1 -> ROOut3/1
  [out3] -> ROOut3/2
  MinMax/1 -> Out1/1

== system c00017M_harness/Eval154 ==
  In1 : Inport
  In2 : Inport  Port=2
  In3 : Inport  Port=3
  In4 : Inport  Port=4
  Data Type Conversion{,1..3} (4 alike) : DataTypeConversion
  Memory{1..4} (4 alike) : Memory  InitialCondition=1
  MinMax : MinMax  Inputs=4
  MinMax{1..4} (4 alike) : MinMax  Inputs=2
  ROOut{1..4} (4 alike) : RelationalOperator  Operator===  OutDataTypeStr=boolean  RndMeth=Simplest
  Out1 : Outport
  wires:
  Data Type Conversion3/1 -> MinMax4/1
  Data Type Conversion2/1 -> MinMax3/1
  Data Type Conversion1/1 -> MinMax2/1
  Data Type Conversion/1 -> MinMax1/1
  MinMax1/1 -> Memory1/1, MinMax/1
  ROOut4/1 -> Data Type Conversion3/1
  MinMax2/1 -> Memory2/1, MinMax/2
  ROOut1/1 -> Data Type Conversion/1
  Memory2/1 -> MinMax2/2
  Memory4/1 -> MinMax4/2
  Memory3/1 -> MinMax3/2
  ROOut2/1 -> Data Type Conversion1/1
  ROOut3/1 -> Data Type Conversion2/1
  MinMax3/1 -> Memory3/1, MinMax/3
  MinMax4/1 -> Memory4/1, MinMax/4
  Memory1/1 -> MinMax1/2
  [out4] -> ROOut4/2
  In4/1 -> ROOut4/1
  [out2] -> ROOut2/2
  In1/1 -> ROOut1/1
  In2/1 -> ROOut2/1
  [out1] -> ROOut1/2
  In3/1 -> ROOut3/1
  [out3] -> ROOut3/2
  MinMax/1 -> Out1/1

== system c00017M_harness/Eval155 ==
  In1 : Inport
  In2 : Inport  Port=2
  In3 : Inport  Port=3
  In4 : Inport  Port=4
  Data Type Conversion{,1..3} (4 alike) : DataTypeConversion
  Memory{1..4} (4 alike) : Memory  InitialCondition=1
  MinMax : MinMax  Inputs=4
  MinMax{1..4} (4 alike) : MinMax  Inputs=2
  ROOut{1..4} (4 alike) : RelationalOperator  Operator===  OutDataTypeStr=boolean  RndMeth=Simplest
  Out1 : Outport
  wires:
  Data Type Conversion3/1 -> MinMax4/1
  Data Type Conversion2/1 -> MinMax3/1
  Data Type Conversion1/1 -> MinMax2/1
  Data Type Conversion/1 -> MinMax1/1
  MinMax1/1 -> Memory1/1, MinMax/1
  ROOut4/1 -> Data Type Conversion3/1
  MinMax2/1 -> Memory2/1, MinMax/2
  ROOut1/1 -> Data Type Conversion/1
  Memory2/1 -> MinMax2/2
  Memory4/1 -> MinMax4/2
  Memory3/1 -> MinMax3/2
  ROOut2/1 -> Data Type Conversion1/1
  ROOut3/1 -> Data Type Conversion2/1
  MinMax3/1 -> Memory3/1, MinMax/3
  MinMax4/1 -> Memory4/1, MinMax/4
  Memory1/1 -> MinMax1/2
  [out4] -> ROOut4/2
  In4/1 -> ROOut4/1
  [out2] -> ROOut2/2
  In1/1 -> ROOut1/1
  In2/1 -> ROOut2/1
  [out1] -> ROOut1/2
  In3/1 -> ROOut3/1
  [out3] -> ROOut3/2
  MinMax/1 -> Out1/1

== system c00017M_harness/Eval156 ==
  In1 : Inport
  In2 : Inport  Port=2
  In3 : Inport  Port=3
  In4 : Inport  Port=4
  Data Type Conversion{,1..3} (4 alike) : DataTypeConversion
  Memory{1..4} (4 alike) : Memory  InitialCondition=1
  MinMax : MinMax  Inputs=4
  MinMax{1..4} (4 alike) : MinMax  Inputs=2
  ROOut{1..4} (4 alike) : RelationalOperator  Operator===  OutDataTypeStr=boolean  RndMeth=Simplest
  Out1 : Outport
  wires:
  Data Type Conversion3/1 -> MinMax4/1
  Data Type Conversion2/1 -> MinMax3/1
  Data Type Conversion1/1 -> MinMax2/1
  Data Type Conversion/1 -> MinMax1/1
  MinMax1/1 -> Memory1/1, MinMax/1
  ROOut4/1 -> Data Type Conversion3/1
  MinMax2/1 -> Memory2/1, MinMax/2
  ROOut1/1 -> Data Type Conversion/1
  Memory2/1 -> MinMax2/2
  Memory4/1 -> MinMax4/2
  Memory3/1 -> MinMax3/2
  ROOut2/1 -> Data Type Conversion1/1
  ROOut3/1 -> Data Type Conversion2/1
  MinMax3/1 -> Memory3/1, MinMax/3
  MinMax4/1 -> Memory4/1, MinMax/4
  Memory1/1 -> MinMax1/2
  [out4] -> ROOut4/2
  In4/1 -> ROOut4/1
  [out2] -> ROOut2/2
  In1/1 -> ROOut1/1
  In2/1 -> ROOut2/1
  [out1] -> ROOut1/2
  In3/1 -> ROOut3/1
  [out3] -> ROOut3/2
  MinMax/1 -> Out1/1

== system c00017M_harness/Eval157 ==
  In1 : Inport
  In2 : Inport  Port=2
  In3 : Inport  Port=3
  In4 : Inport  Port=4
  Data Type Conversion{,1..3} (4 alike) : DataTypeConversion
  Memory{1..4} (4 alike) : Memory  InitialCondition=1
  MinMax : MinMax  Inputs=4
  MinMax{1..4} (4 alike) : MinMax  Inputs=2
  ROOut{1..4} (4 alike) : RelationalOperator  Operator===  OutDataTypeStr=boolean  RndMeth=Simplest
  Out1 : Outport
  wires:
  Data Type Conversion3/1 -> MinMax4/1
  Data Type Conversion2/1 -> MinMax3/1
  Data Type Conversion1/1 -> MinMax2/1
  Data Type Conversion/1 -> MinMax1/1
  MinMax1/1 -> Memory1/1, MinMax/1
  ROOut4/1 -> Data Type Conversion3/1
  MinMax2/1 -> Memory2/1, MinMax/2
  ROOut1/1 -> Data Type Conversion/1
  Memory2/1 -> MinMax2/2
  Memory4/1 -> MinMax4/2
  Memory3/1 -> MinMax3/2
  ROOut2/1 -> Data Type Conversion1/1
  ROOut3/1 -> Data Type Conversion2/1
  MinMax3/1 -> Memory3/1, MinMax/3
  MinMax4/1 -> Memory4/1, MinMax/4
  Memory1/1 -> MinMax1/2
  [out4] -> ROOut4/2
  In4/1 -> ROOut4/1
  [out2] -> ROOut2/2
  In1/1 -> ROOut1/1
  In2/1 -> ROOut2/1
  [out1] -> ROOut1/2
  In3/1 -> ROOut3/1
  [out3] -> ROOut3/2
  MinMax/1 -> Out1/1

== system c00017M_harness/Eval158 ==
  In1 : Inport
  In2 : Inport  Port=2
  In3 : Inport  Port=3
  In4 : Inport  Port=4
  Data Type Conversion{,1..3} (4 alike) : DataTypeConversion
  Memory{1..4} (4 alike) : Memory  InitialCondition=1
  MinMax : MinMax  Inputs=4
  MinMax{1..4} (4 alike) : MinMax  Inputs=2
  ROOut{1..4} (4 alike) : RelationalOperator  Operator===  OutDataTypeStr=boolean  RndMeth=Simplest
  Out1 : Outport
  wires:
  Data Type Conversion3/1 -> MinMax4/1
  Data Type Conversion2/1 -> MinMax3/1
  Data Type Conversion1/1 -> MinMax2/1
  Data Type Conversion/1 -> MinMax1/1
  MinMax1/1 -> Memory1/1, MinMax/1
  ROOut4/1 -> Data Type Conversion3/1
  MinMax2/1 -> Memory2/1, MinMax/2
  ROOut1/1 -> Data Type Conversion/1
  Memory2/1 -> MinMax2/2
  Memory4/1 -> MinMax4/2
  Memory3/1 -> MinMax3/2
  ROOut2/1 -> Data Type Conversion1/1
  ROOut3/1 -> Data Type Conversion2/1
  MinMax3/1 -> Memory3/1, MinMax/3
  MinMax4/1 -> Memory4/1, MinMax/4
  Memory1/1 -> MinMax1/2
  [out4] -> ROOut4/2
  In4/1 -> ROOut4/1
  [out2] -> ROOut2/2
  In1/1 -> ROOut1/1
  In2/1 -> ROOut2/1
  [out1] -> ROOut1/2
  In3/1 -> ROOut3/1
  [out3] -> ROOut3/2
  MinMax/1 -> Out1/1

== system c00017M_harness/Eval159 ==
  In1 : Inport
  In2 : Inport  Port=2
  In3 : Inport  Port=3
  In4 : Inport  Port=4
  Data Type Conversion{,1..3} (4 alike) : DataTypeConversion
  Memory{1..4} (4 alike) : Memory  InitialCondition=1
  MinMax : MinMax  Inputs=4
  MinMax{1..4} (4 alike) : MinMax  Inputs=2
  ROOut{1..4} (4 alike) : RelationalOperator  Operator===  OutDataTypeStr=boolean  RndMeth=Simplest
  Out1 : Outport
  wires:
  Data Type Conversion3/1 -> MinMax4/1
  Data Type Conversion2/1 -> MinMax3/1
  Data Type Conversion1/1 -> MinMax2/1
  Data Type Conversion/1 -> MinMax1/1
  MinMax1/1 -> Memory1/1, MinMax/1
  ROOut4/1 -> Data Type Conversion3/1
  MinMax2/1 -> Memory2/1, MinMax/2
  ROOut1/1 -> Data Type Conversion/1
  Memory2/1 -> MinMax2/2
  Memory4/1 -> MinMax4/2
  Memory3/1 -> MinMax3/2
  ROOut2/1 -> Data Type Conversion1/1
  ROOut3/1 -> Data Type Conversion2/1
  MinMax3/1 -> Memory3/1, MinMax/3
  MinMax4/1 -> Memory4/1, MinMax/4
  Memory1/1 -> MinMax1/2
  [out4] -> ROOut4/2
  In4/1 -> ROOut4/1
  [out2] -> ROOut2/2
  In1/1 -> ROOut1/1
  In2/1 -> ROOut2/1
  [out1] -> ROOut1/2
  In3/1 -> ROOut3/1
  [out3] -> ROOut3/2
  MinMax/1 -> Out1/1

== system c00017M_harness/Eval16 ==
  In1 : Inport
  In2 : Inport  Port=2
  In3 : Inport  Port=3
  In4 : Inport  Port=4
  Data Type Conversion{,1..3} (4 alike) : DataTypeConversion
  Memory{1..4} (4 alike) : Memory  InitialCondition=1
  MinMax : MinMax  Inputs=4
  MinMax{1..4} (4 alike) : MinMax  Inputs=2
  ROOut{1..4} (4 alike) : RelationalOperator  Operator===  OutDataTypeStr=boolean  RndMeth=Simplest
  Out1 : Outport
  wires:
  Data Type Conversion3/1 -> MinMax4/1
  Data Type Conversion2/1 -> MinMax3/1
  Data Type Conversion1/1 -> MinMax2/1
  Data Type Conversion/1 -> MinMax1/1
  MinMax1/1 -> Memory1/1, MinMax/1
  ROOut4/1 -> Data Type Conversion3/1
  MinMax2/1 -> Memory2/1, MinMax/2
  ROOut1/1 -> Data Type Conversion/1
  Memory2/1 -> MinMax2/2
  Memory4/1 -> MinMax4/2
  Memory3/1 -> MinMax3/2
  ROOut2/1 -> Data Type Conversion1/1
  ROOut3/1 -> Data Type Conversion2/1
  MinMax3/1 -> Memory3/1, MinMax/3
  MinMax4/1 -> Memory4/1, MinMax/4
  Memory1/1 -> MinMax1/2
  [out4] -> ROOut4/2
  In4/1 -> ROOut4/1
  [out2] -> ROOut2/2
  In1/1 -> ROOut1/1
  In2/1 -> ROOut2/1
  [out1] -> ROOut1/2
  In3/1 -> ROOut3/1
  [out3] -> ROOut3/2
  MinMax/1 -> Out1/1

== system c00017M_harness/Eval160 ==
  In1 : Inport
  In2 : Inport  Port=2
  In3 : Inport  Port=3
  In4 : Inport  Port=4
  Data Type Conversion{,1..3} (4 alike) : DataTypeConversion
  Memory{1..4} (4 alike) : Memory  InitialCondition=1
  MinMax : MinMax  Inputs=4
  MinMax{1..4} (4 alike) : MinMax  Inputs=2
  ROOut{1..4} (4 alike) : RelationalOperator  Operator===  OutDataTypeStr=boolean  RndMeth=Simplest
  Out1 : Outport
  wires:
  Data Type Conversion3/1 -> MinMax4/1
  Data Type Conversion2/1 -> MinMax3/1
  Data Type Conversion1/1 -> MinMax2/1
  Data Type Conversion/1 -> MinMax1/1
  MinMax1/1 -> Memory1/1, MinMax/1
  ROOut4/1 -> Data Type Conversion3/1
  MinMax2/1 -> Memory2/1, MinMax/2
  ROOut1/1 -> Data Type Conversion/1
  Memory2/1 -> MinMax2/2
  Memory4/1 -> MinMax4/2
  Memory3/1 -> MinMax3/2
  ROOut2/1 -> Data Type Conversion1/1
  ROOut3/1 -> Data Type Conversion2/1
  MinMax3/1 -> Memory3/1, MinMax/3
  MinMax4/1 -> Memory4/1, MinMax/4
  Memory1/1 -> MinMax1/2
  [out4] -> ROOut4/2
  In4/1 -> ROOut4/1
  [out2] -> ROOut2/2
  In1/1 -> ROOut1/1
  In2/1 -> ROOut2/1
  [out1] -> ROOut1/2
  In3/1 -> ROOut3/1
  [out3] -> ROOut3/2
  MinMax/1 -> Out1/1

== system c00017M_harness/Eval161 ==
  In1 : Inport
  In2 : Inport  Port=2
  In3 : Inport  Port=3
  In4 : Inport  Port=4
  Data Type Conversion{,1..3} (4 alike) : DataTypeConversion
  Memory{1..4} (4 alike) : Memory  InitialCondition=1
  MinMax : MinMax  Inputs=4
  MinMax{1..4} (4 alike) : MinMax  Inputs=2
  ROOut{1..4} (4 alike) : RelationalOperator  Operator===  OutDataTypeStr=boolean  RndMeth=Simplest
  Out1 : Outport
  wires:
  Data Type Conversion3/1 -> MinMax4/1
  Data Type Conversion2/1 -> MinMax3/1
  Data Type Conversion1/1 -> MinMax2/1
  Data Type Conversion/1 -> MinMax1/1
  MinMax1/1 -> Memory1/1, MinMax/1
  ROOut4/1 -> Data Type Conversion3/1
  MinMax2/1 -> Memory2/1, MinMax/2
  ROOut1/1 -> Data Type Conversion/1
  Memory2/1 -> MinMax2/2
  Memory4/1 -> MinMax4/2
  Memory3/1 -> MinMax3/2
  ROOut2/1 -> Data Type Conversion1/1
  ROOut3/1 -> Data Type Conversion2/1
  MinMax3/1 -> Memory3/1, MinMax/3
  MinMax4/1 -> Memory4/1, MinMax/4
  Memory1/1 -> MinMax1/2
  [out4] -> ROOut4/2
  In4/1 -> ROOut4/1
  [out2] -> ROOut2/2
  In1/1 -> ROOut1/1
  In2/1 -> ROOut2/1
  [out1] -> ROOut1/2
  In3/1 -> ROOut3/1
  [out3] -> ROOut3/2
  MinMax/1 -> Out1/1

== system c00017M_harness/Eval162 ==
  In1 : Inport
  In2 : Inport  Port=2
  In3 : Inport  Port=3
  In4 : Inport  Port=4
  Data Type Conversion{,1..3} (4 alike) : DataTypeConversion
  Memory{1..4} (4 alike) : Memory  InitialCondition=1
  MinMax : MinMax  Inputs=4
  MinMax{1..4} (4 alike) : MinMax  Inputs=2
  ROOut{1..4} (4 alike) : RelationalOperator  Operator===  OutDataTypeStr=boolean  RndMeth=Simplest
  Out1 : Outport
  wires:
  Data Type Conversion3/1 -> MinMax4/1
  Data Type Conversion2/1 -> MinMax3/1
  Data Type Conversion1/1 -> MinMax2/1
  Data Type Conversion/1 -> MinMax1/1
  MinMax1/1 -> Memory1/1, MinMax/1
  ROOut4/1 -> Data Type Conversion3/1
  MinMax2/1 -> Memory2/1, MinMax/2
  ROOut1/1 -> Data Type Conversion/1
  Memory2/1 -> MinMax2/2
  Memory4/1 -> MinMax4/2
  Memory3/1 -> MinMax3/2
  ROOut2/1 -> Data Type Conversion1/1
  ROOut3/1 -> Data Type Conversion2/1
  MinMax3/1 -> Memory3/1, MinMax/3
  MinMax4/1 -> Memory4/1, MinMax/4
  Memory1/1 -> MinMax1/2
  [out4] -> ROOut4/2
  In4/1 -> ROOut4/1
  [out2] -> ROOut2/2
  In1/1 -> ROOut1/1
  In2/1 -> ROOut2/1
  [out1] -> ROOut1/2
  In3/1 -> ROOut3/1
  [out3] -> ROOut3/2
  MinMax/1 -> Out1/1

== system c00017M_harness/Eval163 ==
  In1 : Inport
  In2 : Inport  Port=2
  In3 : Inport  Port=3
  In4 : Inport  Port=4
  Data Type Conversion{,1..3} (4 alike) : DataTypeConversion
  Memory{1..4} (4 alike) : Memory  InitialCondition=1
  MinMax : MinMax  Inputs=4
  MinMax{1..4} (4 alike) : MinMax  Inputs=2
  ROOut{1..4} (4 alike) : RelationalOperator  Operator===  OutDataTypeStr=boolean  RndMeth=Simplest
  Out1 : Outport
  wires:
  Data Type Conversion3/1 -> MinMax4/1
  Data Type Conversion2/1 -> MinMax3/1
  Data Type Conversion1/1 -> MinMax2/1
  Data Type Conversion/1 -> MinMax1/1
  MinMax1/1 -> Memory1/1, MinMax/1
  ROOut4/1 -> Data Type Conversion3/1
  MinMax2/1 -> Memory2/1, MinMax/2
  ROOut1/1 -> Data Type Conversion/1
  Memory2/1 -> MinMax2/2
  Memory4/1 -> MinMax4/2
  Memory3/1 -> MinMax3/2
  ROOut2/1 -> Data Type Conversion1/1
  ROOut3/1 -> Data Type Conversion2/1
  MinMax3/1 -> Memory3/1, MinMax/3
  MinMax4/1 -> Memory4/1, MinMax/4
  Memory1/1 -> MinMax1/2
  [out4] -> ROOut4/2
  In4/1 -> ROOut4/1
  [out2] -> ROOut2/2
  In1/1 -> ROOut1/1
  In2/1 -> ROOut2/1
  [out1] -> ROOut1/2
  In3/1 -> ROOut3/1
  [out3] -> ROOut3/2
  MinMax/1 -> Out1/1

== system c00017M_harness/Eval164 ==
  In1 : Inport
  In2 : Inport  Port=2
  In3 : Inport  Port=3
  In4 : Inport  Port=4
  Data Type Conversion{,1..3} (4 alike) : DataTypeConversion
  Memory{1..4} (4 alike) : Memory  InitialCondition=1
  MinMax : MinMax  Inputs=4
  MinMax{1..4} (4 alike) : MinMax  Inputs=2
  ROOut{1..4} (4 alike) : RelationalOperator  Operator===  OutDataTypeStr=boolean  RndMeth=Simplest
  Out1 : Outport
  wires:
  Data Type Conversion3/1 -> MinMax4/1
  Data Type Conversion2/1 -> MinMax3/1
  Data Type Conversion1/1 -> MinMax2/1
  Data Type Conversion/1 -> MinMax1/1
  MinMax1/1 -> Memory1/1, MinMax/1
  ROOut4/1 -> Data Type Conversion3/1
  MinMax2/1 -> Memory2/1, MinMax/2
  ROOut1/1 -> Data Type Conversion/1
  Memory2/1 -> MinMax2/2
  Memory4/1 -> MinMax4/2
  Memory3/1 -> MinMax3/2
  ROOut2/1 -> Data Type Conversion1/1
  ROOut3/1 -> Data Type Conversion2/1
  MinMax3/1 -> Memory3/1, MinMax/3
  MinMax4/1 -> Memory4/1, MinMax/4
  Memory1/1 -> MinMax1/2
  [out4] -> ROOut4/2
  In4/1 -> ROOut4/1
  [out2] -> ROOut2/2
  In1/1 -> ROOut1/1
  In2/1 -> ROOut2/1
  [out1] -> ROOut1/2
  In3/1 -> ROOut3/1
  [out3] -> ROOut3/2
  MinMax/1 -> Out1/1

== system c00017M_harness/Eval165 ==
  In1 : Inport
  In2 : Inport  Port=2
  In3 : Inport  Port=3
  In4 : Inport  Port=4
  Data Type Conversion{,1..3} (4 alike) : DataTypeConversion
  Memory{1..4} (4 alike) : Memory  InitialCondition=1
  MinMax : MinMax  Inputs=4
  MinMax{1..4} (4 alike) : MinMax  Inputs=2
  ROOut{1..4} (4 alike) : RelationalOperator  Operator===  OutDataTypeStr=boolean  RndMeth=Simplest
  Out1 : Outport
  wires:
  Data Type Conversion3/1 -> MinMax4/1
  Data Type Conversion2/1 -> MinMax3/1
  Data Type Conversion1/1 -> MinMax2/1
  Data Type Conversion/1 -> MinMax1/1
  MinMax1/1 -> Memory1/1, MinMax/1
  ROOut4/1 -> Data Type Conversion3/1
  MinMax2/1 -> Memory2/1, MinMax/2
  ROOut1/1 -> Data Type Conversion/1
  Memory2/1 -> MinMax2/2
  Memory4/1 -> MinMax4/2
  Memory3/1 -> MinMax3/2
  ROOut2/1 -> Data Type Conversion1/1
  ROOut3/1 -> Data Type Conversion2/1
  MinMax3/1 -> Memory3/1, MinMax/3
  MinMax4/1 -> Memory4/1, MinMax/4
  Memory1/1 -> MinMax1/2
  [out4] -> ROOut4/2
  In4/1 -> ROOut4/1
  [out2] -> ROOut2/2
  In1/1 -> ROOut1/1
  In2/1 -> ROOut2/1
  [out1] -> ROOut1/2
  In3/1 -> ROOut3/1
  [out3] -> ROOut3/2
  MinMax/1 -> Out1/1

== system c00017M_harness/Eval166 ==
  In1 : Inport
  In2 : Inport  Port=2
  In3 : Inport  Port=3
  In4 : Inport  Port=4
  Data Type Conversion{,1..3} (4 alike) : DataTypeConversion
  Memory{1..4} (4 alike) : Memory  InitialCondition=1
  MinMax : MinMax  Inputs=4
  MinMax{1..4} (4 alike) : MinMax  Inputs=2
  ROOut{1..4} (4 alike) : RelationalOperator  Operator===  OutDataTypeStr=boolean  RndMeth=Simplest
  Out1 : Outport
  wires:
  Data Type Conversion3/1 -> MinMax4/1
  Data Type Conversion2/1 -> MinMax3/1
  Data Type Conversion1/1 -> MinMax2/1
  Data Type Conversion/1 -> MinMax1/1
  MinMax1/1 -> Memory1/1, MinMax/1
  ROOut4/1 -> Data Type Conversion3/1
  MinMax2/1 -> Memory2/1, MinMax/2
  ROOut1/1 -> Data Type Conversion/1
  Memory2/1 -> MinMax2/2
  Memory4/1 -> MinMax4/2
  Memory3/1 -> MinMax3/2
  ROOut2/1 -> Data Type Conversion1/1
  ROOut3/1 -> Data Type Conversion2/1
  MinMax3/1 -> Memory3/1, MinMax/3
  MinMax4/1 -> Memory4/1, MinMax/4
  Memory1/1 -> MinMax1/2
  [out4] -> ROOut4/2
  In4/1 -> ROOut4/1
  [out2] -> ROOut2/2
  In1/1 -> ROOut1/1
  In2/1 -> ROOut2/1
  [out1] -> ROOut1/2
  In3/1 -> ROOut3/1
  [out3] -> ROOut3/2
  MinMax/1 -> Out1/1

== system c00017M_harness/Eval167 ==
  In1 : Inport
  In2 : Inport  Port=2
  In3 : Inport  Port=3
  In4 : Inport  Port=4
  Data Type Conversion{,1..3} (4 alike) : DataTypeConversion
  Memory{1..4} (4 alike) : Memory  InitialCondition=1
  MinMax : MinMax  Inputs=4
  MinMax{1..4} (4 alike) : MinMax  Inputs=2
  ROOut{1..4} (4 alike) : RelationalOperator  Operator===  OutDataTypeStr=boolean  RndMeth=Simplest
  Out1 : Outport
  wires:
  Data Type Conversion3/1 -> MinMax4/1
  Data Type Conversion2/1 -> MinMax3/1
  Data Type Conversion1/1 -> MinMax2/1
  Data Type Conversion/1 -> MinMax1/1
  MinMax1/1 -> Memory1/1, MinMax/1
  ROOut4/1 -> Data Type Conversion3/1
  MinMax2/1 -> Memory2/1, MinMax/2
  ROOut1/1 -> Data Type Conversion/1
  Memory2/1 -> MinMax2/2
  Memory4/1 -> MinMax4/2
  Memory3/1 -> MinMax3/2
  ROOut2/1 -> Data Type Conversion1/1
  ROOut3/1 -> Data Type Conversion2/1
  MinMax3/1 -> Memory3/1, MinMax/3
  MinMax4/1 -> Memory4/1, MinMax/4
  Memory1/1 -> MinMax1/2
  [out4] -> ROOut4/2
  In4/1 -> ROOut4/1
  [out2] -> ROOut2/2
  In1/1 -> ROOut1/1
  In2/1 -> ROOut2/1
  [out1] -> ROOut1/2
  In3/1 -> ROOut3/1
  [out3] -> ROOut3/2
  MinMax/1 -> Out1/1

== system c00017M_harness/Eval168 ==
  In1 : Inport
  In2 : Inport  Port=2
  In3 : Inport  Port=3
  In4 : Inport  Port=4
  Data Type Conversion{,1..3} (4 alike) : DataTypeConversion
  Memory{1..4} (4 alike) : Memory  InitialCondition=1
  MinMax : MinMax  Inputs=4
  MinMax{1..4} (4 alike) : MinMax  Inputs=2
  ROOut{1..4} (4 alike) : RelationalOperator  Operator===  OutDataTypeStr=boolean  RndMeth=Simplest
  Out1 : Outport
  wires:
  Data Type Conversion3/1 -> MinMax4/1
  Data Type Conversion2/1 -> MinMax3/1
  Data Type Conversion1/1 -> MinMax2/1
  Data Type Conversion/1 -> MinMax1/1
  MinMax1/1 -> Memory1/1, MinMax/1
  ROOut4/1 -> Data Type Conversion3/1
  MinMax2/1 -> Memory2/1, MinMax/2
  ROOut1/1 -> Data Type Conversion/1
  Memory2/1 -> MinMax2/2
  Memory4/1 -> MinMax4/2
  Memory3/1 -> MinMax3/2
  ROOut2/1 -> Data Type Conversion1/1
  ROOut3/1 -> Data Type Conversion2/1
  MinMax3/1 -> Memory3/1, MinMax/3
  MinMax4/1 -> Memory4/1, MinMax/4
  Memory1/1 -> MinMax1/2
  [out4] -> ROOut4/2
  In4/1 -> ROOut4/1
  [out2] -> ROOut2/2
  In1/1 -> ROOut1/1
  In2/1 -> ROOut2/1
  [out1] -> ROOut1/2
  In3/1 -> ROOut3/1
  [out3] -> ROOut3/2
  MinMax/1 -> Out1/1

== system c00017M_harness/Eval169 ==
  In1 : Inport
  In2 : Inport  Port=2
  In3 : Inport  Port=3
  In4 : Inport  Port=4
  Data Type Conversion{,1..3} (4 alike) : DataTypeConversion
  Memory{1..4} (4 alike) : Memory  InitialCondition=1
  MinMax : MinMax  Inputs=4
  MinMax{1..4} (4 alike) : MinMax  Inputs=2
  ROOut{1..4} (4 alike) : RelationalOperator  Operator===  OutDataTypeStr=boolean  RndMeth=Simplest
  Out1 : Outport
  wires:
  Data Type Conversion3/1 -> MinMax4/1
  Data Type Conversion2/1 -> MinMax3/1
  Data Type Conversion1/1 -> MinMax2/1
  Data Type Conversion/1 -> MinMax1/1
  MinMax1/1 -> Memory1/1, MinMax/1
  ROOut4/1 -> Data Type Conversion3/1
  MinMax2/1 -> Memory2/1, MinMax/2
  ROOut1/1 -> Data Type Conversion/1
  Memory2/1 -> MinMax2/2
  Memory4/1 -> MinMax4/2
  Memory3/1 -> MinMax3/2
  ROOut2/1 -> Data Type Conversion1/1
  ROOut3/1 -> Data Type Conversion2/1
  MinMax3/1 -> Memory3/1, MinMax/3
  MinMax4/1 -> Memory4/1, MinMax/4
  Memory1/1 -> MinMax1/2
  [out4] -> ROOut4/2
  In4/1 -> ROOut4/1
  [out2] -> ROOut2/2
  In1/1 -> ROOut1/1
  In2/1 -> ROOut2/1
  [out1] -> ROOut1/2
  In3/1 -> ROOut3/1
  [out3] -> ROOut3/2
  MinMax/1 -> Out1/1

== system c00017M_harness/Eval17 ==
  In1 : Inport
  In2 : Inport  Port=2
  In3 : Inport  Port=3
  In4 : Inport  Port=4
  Data Type Conversion{,1..3} (4 alike) : DataTypeConversion
  Memory{1..4} (4 alike) : Memory  InitialCondition=1
  MinMax : MinMax  Inputs=4
  MinMax{1..4} (4 alike) : MinMax  Inputs=2
  ROOut{1..4} (4 alike) : RelationalOperator  Operator===  OutDataTypeStr=boolean  RndMeth=Simplest
  Out1 : Outport
  wires:
  Data Type Conversion3/1 -> MinMax4/1
  Data Type Conversion2/1 -> MinMax3/1
  Data Type Conversion1/1 -> MinMax2/1
  Data Type Conversion/1 -> MinMax1/1
  MinMax1/1 -> Memory1/1, MinMax/1
  ROOut4/1 -> Data Type Conversion3/1
  MinMax2/1 -> Memory2/1, MinMax/2
  ROOut1/1 -> Data Type Conversion/1
  Memory2/1 -> MinMax2/2
  Memory4/1 -> MinMax4/2
  Memory3/1 -> MinMax3/2
  ROOut2/1 -> Data Type Conversion1/1
  ROOut3/1 -> Data Type Conversion2/1
  MinMax3/1 -> Memory3/1, MinMax/3
  MinMax4/1 -> Memory4/1, MinMax/4
  Memory1/1 -> MinMax1/2
  [out4] -> ROOut4/2
  In4/1 -> ROOut4/1
  [out2] -> ROOut2/2
  In1/1 -> ROOut1/1
  In2/1 -> ROOut2/1
  [out1] -> ROOut1/2
  In3/1 -> ROOut3/1
  [out3] -> ROOut3/2
  MinMax/1 -> Out1/1

== system c00017M_harness/Eval170 ==
  In1 : Inport
  In2 : Inport  Port=2
  In3 : Inport  Port=3
  In4 : Inport  Port=4
  Data Type Conversion{,1..3} (4 alike) : DataTypeConversion
  Memory{1..4} (4 alike) : Memory  InitialCondition=1
  MinMax : MinMax  Inputs=4
  MinMax{1..4} (4 alike) : MinMax  Inputs=2
  ROOut{1..4} (4 alike) : RelationalOperator  Operator===  OutDataTypeStr=boolean  RndMeth=Simplest
  Out1 : Outport
  wires:
  Data Type Conversion3/1 -> MinMax4/1
  Data Type Conversion2/1 -> MinMax3/1
  Data Type Conversion1/1 -> MinMax2/1
  Data Type Conversion/1 -> MinMax1/1
  MinMax1/1 -> Memory1/1, MinMax/1
  ROOut4/1 -> Data Type Conversion3/1
  MinMax2/1 -> Memory2/1, MinMax/2
  ROOut1/1 -> Data Type Conversion/1
  Memory2/1 -> MinMax2/2
  Memory4/1 -> MinMax4/2
  Memory3/1 -> MinMax3/2
  ROOut2/1 -> Data Type Conversion1/1
  ROOut3/1 -> Data Type Conversion2/1
  MinMax3/1 -> Memory3/1, MinMax/3
  MinMax4/1 -> Memory4/1, MinMax/4
  Memory1/1 -> MinMax1/2
  [out4] -> ROOut4/2
  In4/1 -> ROOut4/1
  [out2] -> ROOut2/2
  In1/1 -> ROOut1/1
  In2/1 -> ROOut2/1
  [out1] -> ROOut1/2
  In3/1 -> ROOut3/1
  [out3] -> ROOut3/2
  MinMax/1 -> Out1/1

== system c00017M_harness/Eval171 ==
  In1 : Inport
  In2 : Inport  Port=2
  In3 : Inport  Port=3
  In4 : Inport  Port=4
  Data Type Conversion{,1..3} (4 alike) : DataTypeConversion
  Memory{1..4} (4 alike) : Memory  InitialCondition=1
  MinMax : MinMax  Inputs=4
  MinMax{1..4} (4 alike) : MinMax  Inputs=2
  ROOut{1..4} (4 alike) : RelationalOperator  Operator===  OutDataTypeStr=boolean  RndMeth=Simplest
  Out1 : Outport
  wires:
  Data Type Conversion3/1 -> MinMax4/1
  Data Type Conversion2/1 -> MinMax3/1
  Data Type Conversion1/1 -> MinMax2/1
  Data Type Conversion/1 -> MinMax1/1
  MinMax1/1 -> Memory1/1, MinMax/1
  ROOut4/1 -> Data Type Conversion3/1
  MinMax2/1 -> Memory2/1, MinMax/2
  ROOut1/1 -> Data Type Conversion/1
  Memory2/1 -> MinMax2/2
  Memory4/1 -> MinMax4/2
  Memory3/1 -> MinMax3/2
  ROOut2/1 -> Data Type Conversion1/1
  ROOut3/1 -> Data Type Conversion2/1
  MinMax3/1 -> Memory3/1, MinMax/3
  MinMax4/1 -> Memory4/1, MinMax/4
  Memory1/1 -> MinMax1/2
  [out4] -> ROOut4/2
  In4/1 -> ROOut4/1
  [out2] -> ROOut2/2
  In1/1 -> ROOut1/1
  In2/1 -> ROOut2/1
  [out1] -> ROOut1/2
  In3/1 -> ROOut3/1
  [out3] -> ROOut3/2
  MinMax/1 -> Out1/1
